simulink model "Bai04"  (R2023b)
settings: Solver=VariableStepAuto  StartTime=0.0  StopTime=1  RelTol=1e-3
libraries: commdigbbndpm3 x1
settings Model: Creator=Trung  LastModifiedBy=Trung

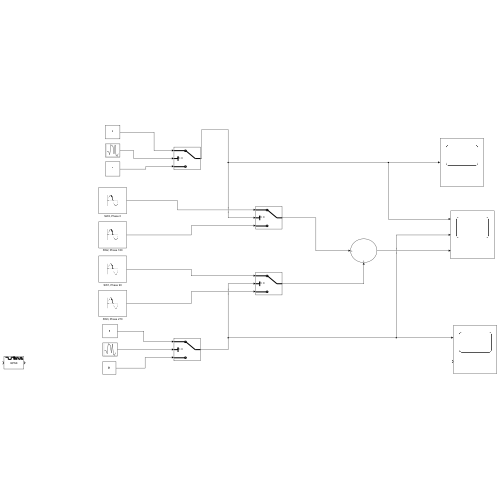
[thumbnail: Simulink's stored preview of the top-level diagram]
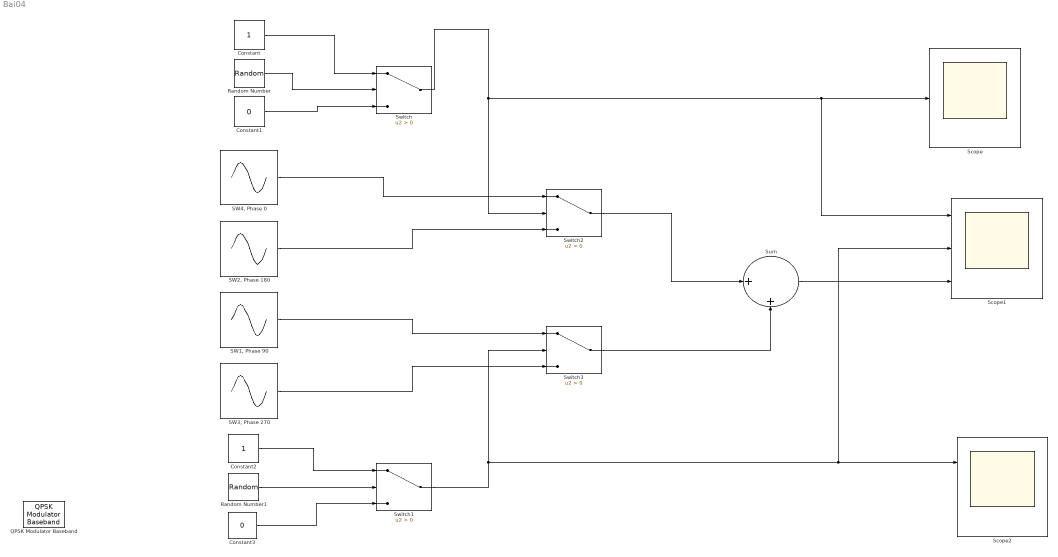
== system Bai04 ==
  Constant : Constant
  Constant1 : Constant  Value=0
  Constant2 : Constant
  Constant3 : Constant  Value=0
  QPSK Modulator Baseband : commdigbbndpm3/QPSK Modulator Baseband  InType=Integer  Enc=Gray  Ph=pi/4  outDtype=double  outWordLen=16  outUDDataType=sfix(16)  outFracLenMode=Best precision  outFracLen=15  outDataTypeStr=double  outLastDataTypeStr=double
      settings: LibrarySourceBlock=|
      | commhdldigbbndpm/QPSK
      | Modulator
      | Baseband
  Random Number : RandomNumber  Seed=20  SampleTime=0.1
  Random Number1 : RandomNumber  Seed=30  SampleTime=0.1
  "SW1, Phase 90" : Sin  Frequency=40 * pi  Phase=pi/2  SampleTime=0.0001
  "SW2, Phase 180" : Sin  Frequency=40 * pi  Phase=pi  SampleTime=0.0001
  "SW3, Phase 270" : Sin  Frequency=40 * pi  Phase=3/2*pi  SampleTime=0.0001
  "SW4, Phase 0" : Sin  Frequency=40 * pi  SampleTime=0.0001
  Scope : Scope
  Scope1 : Scope  NumInputPorts=3
  Scope2 : Scope  NumInputPorts=2
  Sum : Sum  Inputs=|++
  Switch{,1..3} (4 alike) : Switch  Criteria=u2 > Threshold  SaturateOnIntegerOverflow=off  InputSameDT=off
  wires:
  Random Number/1 -> Switch/2
  Constant2/1 -> Switch1/1
  Random Number1/1 -> Switch1/2
  Constant3/1 -> Switch1/3
  Constant/1 -> Switch/1
  Constant1/1 -> Switch/3
  Switch/1 -> Switch2/2, Scope1/1, Scope/1
  "SW4, Phase 0"/1 -> Switch2/1
  "SW2, Phase 180"/1 -> Switch2/3
  "SW1, Phase 90"/1 -> Switch3/1
  "SW3, Phase 270"/1 -> Switch3/3
  Switch1/1 -> Scope1/2, Scope2/1, Switch3/2
  Switch2/1 -> Sum/1
  Switch3/1 -> Sum/2
  Sum/1 -> Scope1/3
